simulink model "LCM_Test"  (R2023a)
settings: Solver=FixedStepAuto  StartTime=0.0  StopTime=inf  FixedStep=0.01  RelTol=1e-3
settings Model: PacingRate=100  Creator=XboxX  LastModifiedBy=XboxX

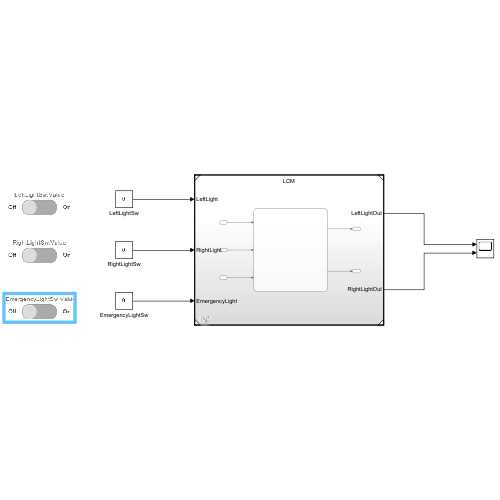
[thumbnail: Simulink's stored preview of the top-level diagram]
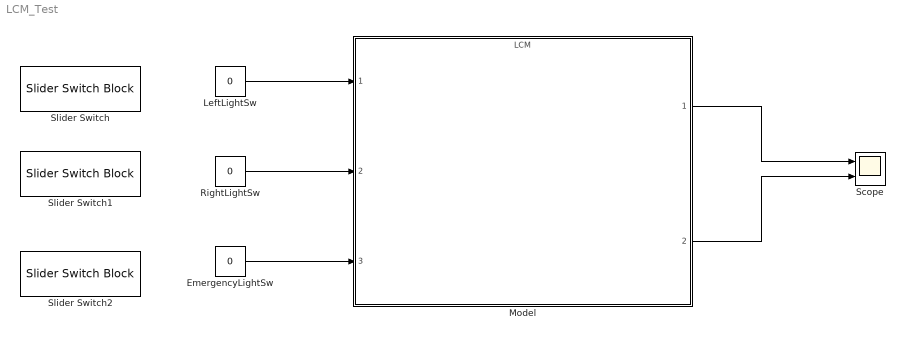
== system LCM_Test ==
  EmergencyLightSw : Constant  Value=0  OutDataTypeStr=boolean
  LeftLightSw : Constant  Value=0  OutDataTypeStr=boolean
  Model : ModelReference  ModelNameDialog=LCM.slx  SimulationMode=Normal  ModelReferenceVersion=1.15
  RightLightSw : Constant  Value=0  OutDataTypeStr=boolean
  Scope : Scope  NumInputPorts=2
  Slider Switch : SliderSwitchBlock
      settings: Values={{'Off', 'On'}, [0 1]}
  Slider Switch1 : SliderSwitchBlock
      settings: Values={{'Off', 'On'}, [0 1]}
  Slider Switch2 : SliderSwitchBlock
      settings: Values={{'Off', 'On'}, [0 1]}
  wires:
  LeftLightSw/1 -> Model/1
  RightLightSw/1 -> Model/2
  EmergencyLightSw/1 -> Model/3
  Model/1 -> Scope/1
  Model/2 -> Scope/2
